simulink model "MDL_example01"  (Simulink 6.1)
settings: Solver=FixedStepDiscrete  SolverMode=SingleTasking  StartTime=0.0  StopTime=N  FixedStep=1  RelTol=1e-3
settings Model: LastModifiedBy=ybstrong
settings DebuggingCC: SolverPrmCheckMsg=warning

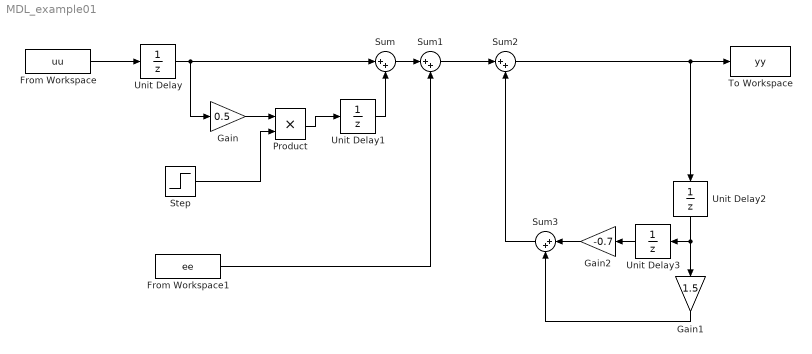
== system MDL_example01 ==
  From Workspace : FromWorkspace  VariableName=uu  SampleTime=1
  From Workspace1 : FromWorkspace  VariableName=ee  SampleTime=1
  Gain : Gain  Gain=0.5
  Gain1 : Gain  Orientation=down  Gain=1.5
  Gain2 : Gain  Orientation=left  Gain=-0.7
  Product : Product  RndMeth=Zero
  Step : Step  Time=50  Before=1  After=0.5  SampleTime=1
  Sum : Sum  Inputs=|++
  Sum1 : Sum  Inputs=|++
  Sum2 : Sum  Inputs=|++
  Sum3 : Sum  Orientation=left  Inputs=|++
  To Workspace : ToWorkspace  VariableName=yy  SampleTime=-1  SaveFormat=Array
  Unit Delay : UnitDelay
  Unit Delay1 : UnitDelay
  Unit Delay2 : UnitDelay  Orientation=down
  Unit Delay3 : UnitDelay  Orientation=left
  wires:
  From Workspace/1 -> Unit Delay/1
  Unit Delay/1 -> Sum/1, Gain/1
  Unit Delay1/1 -> Sum/2
  Gain/1 -> Product/1
  Sum/1 -> Sum1/1
  From Workspace1/1 -> Sum1/2
  Sum1/1 -> Sum2/1
  Sum2/1 -> To Workspace/1, Unit Delay2/1
  Unit Delay2/1 -> Gain1/1, Unit Delay3/1
  Gain1/1 -> Sum3/2
  Unit Delay3/1 -> Gain2/1
  Sum3/1 -> Sum2/2
  Gain2/1 -> Sum3/1
  Product/1 -> Unit Delay1/1
  Step/1 -> Product/2
